simulink model "FinalModel"  (R2022a)
settings: Solver=VariableStepAuto  StartTime=0.0  StopTime=1  RelTol=1e-3
model workspace (MAT data in the model file):
  a = 50
  x = 100
undefined symbols (not defined in the file): gray
libraries: visionsources x2
settings Model: Creator=Dell  LastModifiedBy=Dell

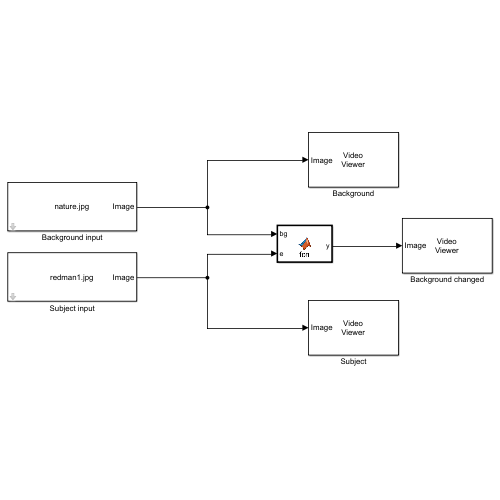
[thumbnail: Simulink's stored preview of the top-level diagram]
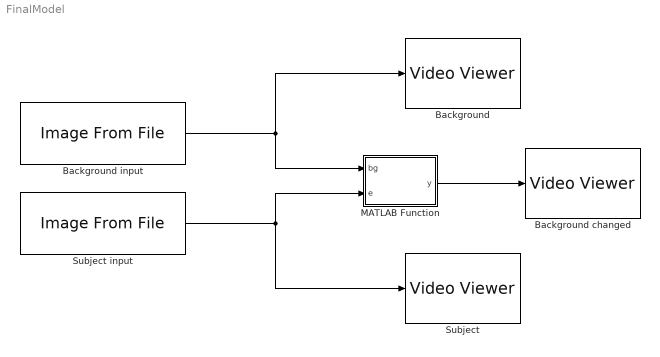
== system FinalModel ==
  Background : VideoViewer  FigPos=[843.4 553.2 539.2 344]
  Background changed : VideoViewer  colormapValue=gray(256)  FigPos=[1 862 1536 764]
  Background input : visionsources/Image From File  Tag=vipblks_nd  FileName=F:\LTTS\project\nature.jpg  Ts=inf  imagePorts=One multidimensional signal  OutPortLabels=R|G|B  ImageDataType=Inherit from input image  sdImageDataType=uint(8)  Signed=on  WordLength=16  FractionLengthMode=User-defined  FractionLength=15
  MATLAB Function : MATLAB Function  TreatAsAtomicUnit=on
  Subject : VideoViewer  FigPos=[9.8 625.2 490.4 371.2]
  Subject input : visionsources/Image From File  Tag=vipblks_nd  FileName=F:\LTTS\project\redman1.jpg  Ts=inf  imagePorts=One multidimensional signal  OutPortLabels=R|G|B  ImageDataType=Inherit from input image  sdImageDataType=uint(8)  Signed=on  WordLength=16  FractionLengthMode=User-defined  FractionLength=15
  wires:
  Background input/1 -> Background/1, MATLAB Function/1(bg)
  MATLAB Function/1(y) -> Background changed/1
  Subject input/1 -> MATLAB Function/2(e), Subject/1

== matlab function FinalModel/MATLAB Function ==
  data: bg input; y output; e input
function y = fcn(bg, e)


% clc
% clear all
% close all
% warning off
% e=imread("redman2.png");
% figure;
% imshow(e);
% bg=imread('road.jpg');


function [BW,maskedRGBImage] = createMask(RGB)
%createMask  Threshold RGB image using auto-generated code from colorThresholder app.
%  [BW,MASKEDRGBIMAGE] = createMask(RGB) thresholds image RGB using
%  auto-generated code from the colorThresholder app. The colorspace and
%  range for each channel of the colorspace were set within the app. The
%  segmentation mask is returned in BW, and a composite of the mask and
%  original RGB images is returned in maskedRGBImage.

% Auto-generated by colorThresholder app on 13-Aug-2020
%------------------------------------------------------


% Convert RGB image to chosen color space
I = rgb2hsv(RGB);

% Define thresholds for channel 1 based on histogram settings
channel1Min = 0.196;
channel1Max = 0.000;

% Define thresholds for channel 2 based on histogram settings
channel2Min = 0.000;
channel2Max = 0.236;

% Define thresholds for channel 3 based on histogram settings
channel3Min = 0.322;
channel3Max = 1.000;

% Create mask based on chosen histogram thresholds
sliderBW = ( (I(:,:,1) >= channel1Min) | (I(:,:,1) <= channel1Max) ) & ...
    (I(:,:,2) >= channel2Min ) & (I(:,:,2) <= channel2Max) & ...
    (I(:,:,3) >= channel3Min ) & (I(:,:,3) <= channel3Max);
BW = sliderBW;

% Invert mask
BW = ~BW;

% Initialize output masked image based on input image.
maskedRGBImage = RGB;

% Set background pixels where BW is false to zero.
maskedRGBImage(repmat(~BW,[1 1 3])) = 0;



% [baseFileName, folder] = uigetfile('*.jpg','Select The Image'); 
% fullFileName = fullfile(folder, baseFileName);
% bg = imread(fullFileName);

% figure;
% imshow(bg);
end

[r c b]=size(e);
gm=imresize(bg,[r c]);
mkdir=createMask(e);
gs=gm.*uint8(~mkdir);
% figure;
% imshow(gs);
% subplot(1,2,1);
% % imshow(e);
% subplot(1,2,2);
gm=bg;
y=(gs+e.*uint8(mkdir));
end
